simulink model "Lab7_pkt1"  (R2017a)
settings: Solver=VariableStepAuto  StartTime=0.0  StopTime=10.0  MaxStep=0.1  RelTol=1e-3
values from neighbouring files (symbols this model uses):
  t0 = (k - b)/a    [Lab4.m]    (also in Lab7.m = 71.2)
libraries: cstblocks x2
settings Model: Creator=ishiguro  LastModifiedBy=ishiguro

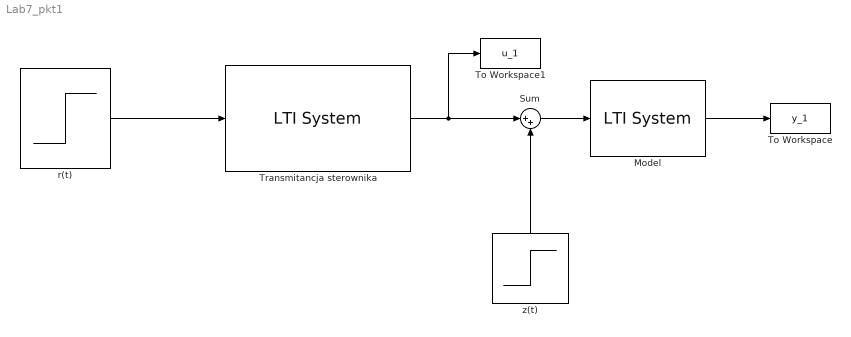
== system Lab7_pkt1 ==
  Model : cstblocks/LTI System  sys=K  IC=[]
  Sum : Sum  Inputs=|++
  To Workspace : ToWorkspace  VariableName=y_1  SampleTime=-1
  To Workspace1 : ToWorkspace  VariableName=u_1  SampleTime=-1
  Transmitancja sterownika : cstblocks/LTI System  sys=Kff  IC=[]
  r(t) : Step  Time=0  SampleTime=0
  z(t) : Step  Time=t0  SampleTime=0
  wires:
  r(t)/1 -> Transmitancja sterownika/1
  z(t)/1 -> Sum/2
  Sum/1 -> Model/1
  Model/1 -> To Workspace/1
  Transmitancja sterownika/1 -> To Workspace1/1, Sum/1
